simulink model "DCmotor02"  (R2019b)
settings: Solver=ode45  StartTime=0.0  StopTime=0.5  MaxStep=1e-6  RelTol=1e-3
undefined symbols (not defined in the file): IaN, Ki_cur, Ki_spd, Kp_cur, Kp_spd, nN, TA, TB, Tfi, Tfn, TN
libraries: powerlib x11, simulink x1
Description:
  | H桥双极式直流电机开环
settings Model: Creator=DELL  LastModifiedBy=Inspiron
settings DataIOCC: ReturnWorkspaceOutputs=off
settings DebuggingCC: ArithmeticOperatorsInVariantConditions=warning
settings SFSimCC: SimUseLocalCustomCode=off  CustomCodeUndefinedFunction=UseInterfaceOnly
settings RTWCC: RTWUseLocalCustomCode=off
settings CodeAppCC: StateflowObjectComments=on
settings SimscapeCC: SimscapeNormalizeSystem=off

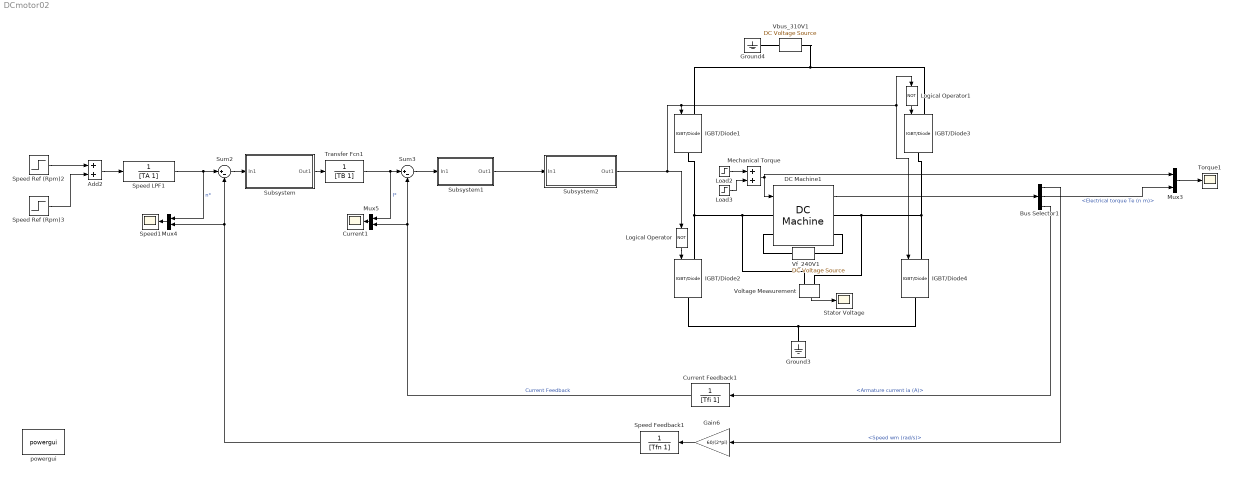
== system DCmotor02 ==
  Add2 : Sum
  Bus Selector1 : BusSelector  OutputSignals=Speed wm (rad/s),Electrical torque Te (n m),Armature current ia (A)
  Current Feedback1 : TransferFcn  Denominator=[Tfi 1]
  Current1 : Scope
  DC Machine1 : powerlib/Machines/DC Machine  PresetModel=No  MechanicalLoad=Torque TL  FieldType=Wound  ShowDetailedParameters=on  MeasurementBus=off  RLa="[ 0.6  0.012]"  RLf="[ 240  120]"  Laf=1.8  MachineConstant=Torque constant (N.m/A)  Ke=1.8  Kt=1.8  J=0.05  Bm=0  Tf=0  w0=1  Ifinit=1  TsPowergui=0  TsBlock=-1
      settings: SourceProductName=Simscape Electrical
  Gain6 : Gain  Gain=60/(2*pi)
  Ground3 : powerlib/Elements/Ground  LConnTagsString=a
      settings: SourceProductName=Simscape Electrical
  Ground4 : powerlib/Elements/Ground  LConnTagsString=a
      settings: SourceProductName=Simscape Electrical
  IGBT/Diode{1..4} (4 alike) : powerlib/Power Electronics/IGBT//Diode  Ron=1e-3  Rs=1e5  Cs=inf  Measurements=off
      settings: SourceProductName=Simscape Electrical
  Load2 : Step  Time=0.4  After=TN  SampleTime=0
  Load3 : Step  Time=0.6  After=-0.2*TN  SampleTime=0
  Logical Operator : Logic  Operator=NOT  AllPortsSameDT=off  OutDataTypeStr=boolean
  Logical Operator1 : Logic  Operator=NOT  AllPortsSameDT=off  OutDataTypeStr=boolean
  Mechanical Torque : Sum
  Mux3 : Mux  Inputs=2
  Mux4 : Mux  Inputs=2
  Mux5 : Mux  Inputs=2
  Speed Feedback1 : TransferFcn  Denominator=[Tfn 1]
  Speed LPF1 : TransferFcn  Denominator=[TA 1]
  Speed Ref (Rpm)2 : Step  Time=0.2  After=0.8*nN  SampleTime=0
  Speed Ref (Rpm)3 : Step  Time=0.8  After=-0.3*nN  SampleTime=0  VectorParams1D=off
  Speed1 : Scope
  Stator Voltage : Scope
  Subsystem : Subsystem
  Subsystem1 : Subsystem
  Subsystem2 : Subsystem
  Sum2 : Sum  Inputs=|+-
  Sum3 : Sum  Inputs=|+-
  Torque1 : Scope
  Transfer Fcn1 : TransferFcn  Denominator=[TB 1]
  Vbus_310V1 : powerlib/Electrical Sources/DC Voltage Source  Amplitude=310  Measurements=None
      settings: SourceProductName=Simscape Electrical
  Vf_240V1 : powerlib/Electrical Sources/DC Voltage Source  Amplitude=240  Measurements=None
      settings: SourceProductName=Simscape Electrical
  Voltage Measurement : powerlib/Measurements/Voltage Measurement  PhasorSimulation=off  OutputType=Complex  PSBequivalent=0
      settings: SourceProductName=Simscape Electrical
  powergui : powerlib/powergui  Priority=1  SimulationMode=Continuous  SampleTime=50e-6  frequency=60  Iterations=50  frequencyindice=0  Pbase=100e6  ErrMax=1e-4  UnitsV=kV  UnitsW=MW  buscounter=0  FunctionMessages=off  echomessages=off  EnableUseOfTLC=off  CurrentSourceSwitches=on  DisableSnubberDevices=off  DisableRonSwitches=off  DisableVfSwitches=off  DisplayEquations=off  AutomaticDiscreteSolvers=off  SolverType=Tustin/Backward Euler (TBE)  Interpol=off  ExternalGateDelay=off  methode=off  Ts=10  x0status=blocks  SPID=off  SwTol=0  HookPort=off  NonlinearTolerance=1e-4  nMaxIteration=100  ContinueOnMaxIteration=off  RestoreLinks=warning  ResistiveCurrentMeasurement=off  Frange=[0:2:500]  Ylog=off  Xlog=on  ShowGrid=off  save=off  variable=ZData  structure=0  ZoomFFT=off  StartTime=0.0  cycles=1  DisplayStyle=1  fundamental=60  FreqAxis=off  MaxFrequency=1000  frequencyindicesteady=1  RmsSteady=1  display=off
      settings: SourceProductName=Simscape Electrical
  wires:
  Current Feedback1/1 -> Sum3/2, Mux5/2  "Current Feedback"
  Bus Selector1/3 -> Current Feedback1/1  "<Armature current ia (A)>"
  Speed Ref (Rpm)2/1 -> Add2/1
  Logical Operator1/1 -> IGBT/Diode3/1
  Speed Ref (Rpm)3/1 -> Add2/2
  Sum2/1 -> Subsystem/1(In1)
  Load3/1 -> Mechanical Torque/2
  Load2/1 -> Mechanical Torque/1
  Mux3/1 -> Torque1/1
  Mechanical Torque/1 -> DC Machine1/1, Mux3/1
  Transfer Fcn1/1 -> Sum3/1, Mux5/1  "I*"
  Subsystem2/1(Out1) -> Logical Operator/1, IGBT/Diode4/1, Logical Operator1/1, IGBT/Diode1/1
  Logical Operator/1 -> IGBT/Diode2/1
  Mux5/1 -> Current1/1
  DC Machine1/1 -> Bus Selector1/1
  Add2/1 -> Speed LPF1/1
  Gain6/1 -> Speed Feedback1/1
  Subsystem/1(Out1) -> Transfer Fcn1/1
  Bus Selector1/2 -> Mux3/2  "<Electrical torque Te (n m)>"
  Voltage Measurement/1 -> Stator Voltage/1
  Bus Selector1/1 -> Gain6/1  "<Speed wm (rad/s)>"
  Speed Feedback1/1 -> Sum2/2, Mux4/2
  Mux4/1 -> Speed1/1
  Speed LPF1/1 -> Sum2/1, Mux4/1  "n*"
  Sum3/1 -> Subsystem1/1(In1)
  Subsystem1/1(Out1) -> Subsystem2/1(In1)
  connections:
  Vbus_310V1/LConn1 -- Ground4/LConn1
  Vbus_310V1/RConn1 -- IGBT/Diode3/LConn1 -- IGBT/Diode1/LConn1
  IGBT/Diode2/LConn1 -- DC Machine1/LConn1 -- Voltage Measurement/LConn1 -- IGBT/Diode1/RConn1
  IGBT/Diode2/RConn1 -- Ground3/LConn1 -- IGBT/Diode4/RConn1
  IGBT/Diode3/RConn1 -- DC Machine1/RConn1 -- Voltage Measurement/LConn2 -- IGBT/Diode4/LConn1
  Vf_240V1/RConn1 -- DC Machine1/LConn2
  Vf_240V1/LConn1 -- DC Machine1/RConn2

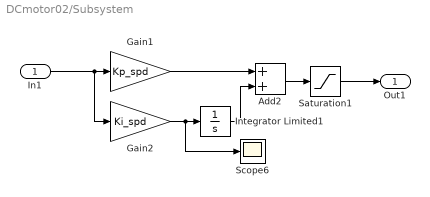
== system DCmotor02/Subsystem ==
  In1 : Inport
  Add2 : Sum
  Gain1 : Gain  Gain=Kp_spd
  Gain2 : Gain  Gain=Ki_spd
  Integrator Limited1 : Integrator  LimitOutput=on  UpperSaturationLimit=2*IaN  LowerSaturationLimit=0
  Saturation1 : Saturate  UpperLimit=2*IaN  LowerLimit=-2*IaN
  Scope6 : Scope
  Out1 : Outport
  wires:
  Gain1/1 -> Add2/1
  In1/1 -> Gain1/1, Gain2/1
  Saturation1/1 -> Out1/1
  Gain2/1 -> Scope6/1, Integrator Limited1/1
  Integrator Limited1/1 -> Add2/2
  Add2/1 -> Saturation1/1

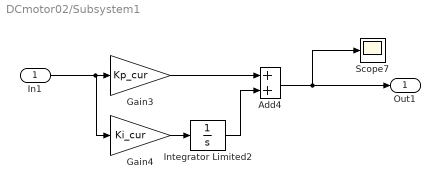
== system DCmotor02/Subsystem1 ==
  In1 : Inport
  Add4 : Sum
  Gain3 : Gain  Gain=Kp_cur
  Gain4 : Gain  Gain=Ki_cur
  Integrator Limited2 : Integrator  LimitOutput=on  UpperSaturationLimit=2*IaN  LowerSaturationLimit=0
  Scope7 : Scope
  Out1 : Outport
  wires:
  Gain3/1 -> Add4/1
  Gain4/1 -> Integrator Limited2/1
  Add4/1 -> Scope7/1, Out1/1
  Integrator Limited2/1 -> Add4/2
  In1/1 -> Gain4/1, Gain3/1

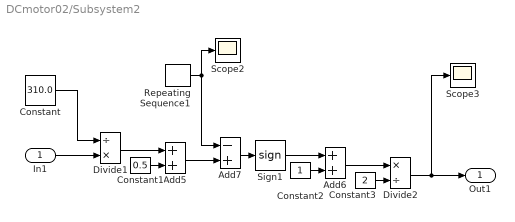
== system DCmotor02/Subsystem2 ==
  In1 : Inport
  Add5 : Sum
  Add6 : Sum
  Add7 : Sum  Inputs=-+
  Constant : Constant  Value=310.0
  Constant1 : Constant  Value=0.5
  Constant2 : Constant
  Constant3 : Constant  Value=2
  Divide1 : Product  Inputs=/*
  Divide2 : Product  Inputs=*/
  Repeating Sequence1 : simulink/Sources/Repeating Sequence  rep_seq_t=[0 100e-6 200e-6]  rep_seq_y=[0 1 0]
  Scope2 : Scope
  Scope3 : Scope
  Sign1 : Signum
  Out1 : Outport
  wires:
  Constant3/1 -> Divide2/2
  Add5/1 -> Add7/2
  Constant1/1 -> Add5/2
  Constant2/1 -> Add6/2
  Divide2/1 -> Out1/1, Scope3/1
  Divide1/1 -> Add5/1
  Add6/1 -> Divide2/1
  Add7/1 -> Sign1/1
  Sign1/1 -> Add6/1
  Repeating Sequence1/1 -> Scope2/1, Add7/1
  Constant/1 -> Divide1/1
  In1/1 -> Divide1/2
